simulink model "task_5_f_lin"  (R2024a)
settings: Solver=VariableStepAuto  StartTime=0.0  StopTime=15  MaxStep=1e-3  RelTol=1e-3
undefined symbols (not defined in the file or in its folder): A, B, C, D, Gamma_f, K, Kf, w_0, x_0, Yf
settings Model: Creator=user  LastModifiedBy=user

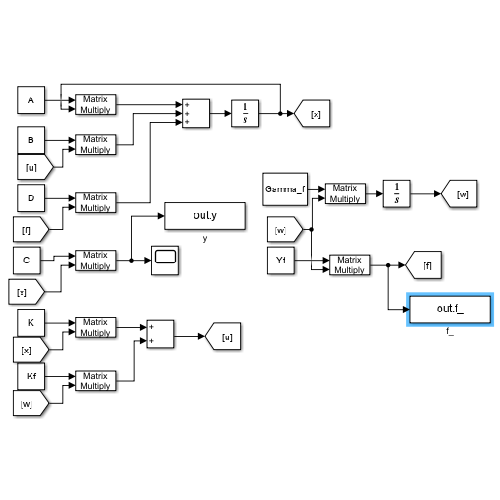
[thumbnail: Simulink's stored preview of the top-level diagram]
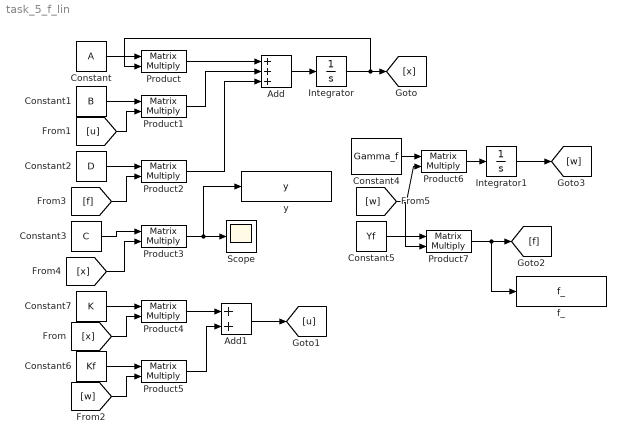
== system task_5_f_lin ==
  Add : Sum  Inputs=+++
  Add1 : Sum
  Constant : Constant  Value=A  VectorParams1D=off
  Constant1 : Constant  Value=B  VectorParams1D=off
  Constant2 : Constant  Value=D  VectorParams1D=off
  Constant3 : Constant  Value=C  VectorParams1D=off
  Constant4 : Constant  Value=Gamma_f  VectorParams1D=off
  Constant5 : Constant  Value=Yf  VectorParams1D=off
  Constant6 : Constant  Value=Kf  VectorParams1D=off
  Constant7 : Constant  Value=K  VectorParams1D=off
  Integrator : Integrator  InitialCondition=x_0
  Integrator1 : Integrator  InitialCondition=w_0
  Product{,1..7} (8 alike) : Product  Multiplication=Matrix(*)
  Scope : Scope
  f_ : ToWorkspace  VariableName=f_  SaveFormat=Timeseries  SampleTime=-1
  y : ToWorkspace  VariableName=y  SaveFormat=Timeseries  SampleTime=-1
  wires:
  Constant/1 -> Product/1
  Add/1 -> Integrator/1
  Product/1 -> Add/1
  Integrator/1 -> [x], Product/2
  Constant7/1 -> Product4/1
  Constant6/1 -> Product5/1
  Product4/1 -> Add1/1
  Product5/1 -> Add1/2
  Add1/1 -> [u]
  [x] -> Product4/2
  Constant2/1 -> Product2/1
  [f] -> Product2/2
  Product2/1 -> Add/3
  Constant1/1 -> Product1/1
  [u] -> Product1/2
  Product1/1 -> Add/2
  Constant3/1 -> Product3/1
  [x] -> Product3/2
  Product3/1 -> y/1, Scope/1
  Constant4/1 -> Product6/1
  Product6/1 -> Integrator1/1
  Integrator1/1 -> [w]
  [w] -> Product7/2, Product6/2
  Constant5/1 -> Product7/1
  Product7/1 -> f_/1, [f]
  [w] -> Product5/2
